simulink model "MDAC3p5bit"  (R2019b)
settings: Solver=VariableStepAuto  StartTime=0.0  StopTime=100.0  RelTol=1e-3
values from neighbouring files (symbols this model uses):
  ts = 1/fs    (= 1)    [launch_pipeline_16ibt.m]
libraries: simulink x1
settings Model: Creator=86184  LastModifiedBy=86184

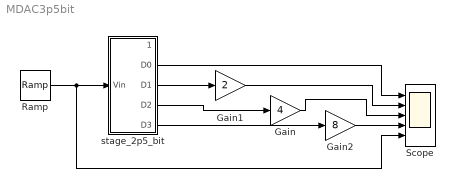
== system MDAC3p5bit ==
  Gain : Gain  Gain=4
  Gain1 : Gain  Gain=2
  Gain2 : Gain  Gain=8
  Ramp : simulink/Sources/Ramp  slope=0.1  start=0  InitialOutput=-5
  Scope : Scope  NumInputPorts=5
  stage_2p5_bit : Subsystem
  wires:
  Ramp/1 -> Scope/5, stage_2p5_bit/1(Vin)
  stage_2p5_bit/2(D0) -> Scope/1
  stage_2p5_bit/3(D1) -> Gain1/1
  stage_2p5_bit/4(D2) -> Gain/1
  Gain1/1 -> Scope/2
  Gain/1 -> Scope/3
  stage_2p5_bit/5(D3) -> Gain2/1
  Gain2/1 -> Scope/4

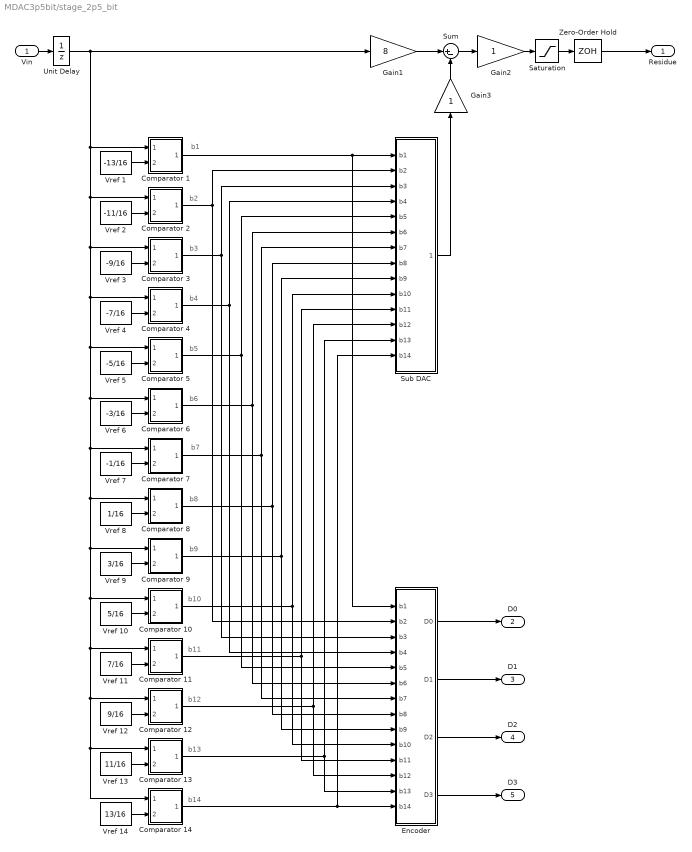
== system MDAC3p5bit/stage_2p5_bit ==
  note: b2
  note: b1
  note: b3
  note: b4
  note: b5
  note: b6
  note: b10
  note: b7
  note: b9
  note: b8
  note: b12
  note: b11
  note: b13
  note: b14
  Vin : Inport
  Comparator 1 : Subsystem
  Comparator 10 : Subsystem
  Comparator 11 : Subsystem
  Comparator 12 : Subsystem
  Comparator 13 : Subsystem
  Comparator 14 : Subsystem
  Comparator 2 : Subsystem
  Comparator 3 : Subsystem
  Comparator 4 : Subsystem
  Comparator 5 : Subsystem
  Comparator 6 : Subsystem
  Comparator 7 : Subsystem
  Comparator 8 : Subsystem
  Comparator 9 : Subsystem
  Encoder : Subsystem
  Gain1 : Gain  Gain=8
  Gain2 : Gain
  Gain3 : Gain
  Saturation : Saturate  UpperLimit=1  LowerLimit=-1
  Sub DAC : Subsystem
  Sum : Sum  Inputs=|+-
  Unit Delay : UnitDelay  SampleTime=-1  HasFrameUpgradeWarning=on
  Vref 1 : Constant  Value=-13/16
  Vref 10 : Constant  Value=5/16
  Vref 11 : Constant  Value=7/16
  Vref 12 : Constant  Value=9/16
  Vref 13 : Constant  Value=11/16
  Vref 14 : Constant  Value=13/16
  Vref 2 : Constant  Value=-11/16
  Vref 3 : Constant  Value=-9/16
  Vref 4 : Constant  Value=-7/16
  Vref 5 : Constant  Value=-5/16
  Vref 6 : Constant  Value=-3/16
  Vref 7 : Constant  Value=-1/16
  Vref 8 : Constant  Value=1/16
  Vref 9 : Constant  Value=3/16
  Zero-Order Hold : ZeroOrderHold  SampleTime=ts
  Residue : Outport
  D0 : Outport  Port=2
  D1 : Outport  Port=3
  D2 : Outport  Port=4
  D3 : Outport  Port=5
  wires:
  Vref 1/1 -> Comparator 1/2(Vref)
  Sub DAC/1(Vdac) -> Gain3/1
  Gain1/1 -> Sum/1
  Gain3/1 -> Sum/2
  Sum/1 -> Gain2/1
  Saturation/1 -> Zero-Order Hold/1
  Zero-Order Hold/1 -> Residue/1
  Gain2/1 -> Saturation/1
  Vref 2/1 -> Comparator 2/2(Vref)
  Vin/1 -> Unit Delay/1
  Vref 3/1 -> Comparator 3/2(Vref)
  Vref 4/1 -> Comparator 4/2(Vref)
  Vref 5/1 -> Comparator 5/2(Vref)
  Vref 6/1 -> Comparator 6/2(Vref)
  Unit Delay/1 -> Comparator 14/1(Vin), Comparator 13/1(Vin), Comparator 12/1(Vin), Comparator 11/1(Vin), Comparator 10/1(Vin), Comparator 9/1(Vin), Comparator 8/1(Vin), Comparator 7/1(Vin), Comparator 6/1(Vin), Comparator 5/1(Vin), Comparator 4/1(Vin), Comparator 3/1(Vin), Comparator 2/1(Vin), Comparator 1/1(Vin), Gain1/1
  Vref 11/1 -> Comparator 11/2(Vref)
  Vref 9/1 -> Comparator 9/2(Vref)
  Vref 7/1 -> Comparator 7/2(Vref)
  Vref 12/1 -> Comparator 12/2(Vref)
  Vref 10/1 -> Comparator 10/2(Vref)
  Vref 8/1 -> Comparator 8/2(Vref)
  Vref 14/1 -> Comparator 14/2(Vref)
  Vref 13/1 -> Comparator 13/2(Vref)
  Comparator 1/1(Out) -> Sub DAC/1(b1), Encoder/1(b1)
  Comparator 2/1(Out) -> Encoder/2(b2), Sub DAC/2(b2)
  Comparator 3/1(Out) -> Encoder/3(b3), Sub DAC/3(b3)
  Comparator 4/1(Out) -> Encoder/4(b4), Sub DAC/4(b4)
  Comparator 5/1(Out) -> Encoder/5(b5), Sub DAC/5(b5)
  Comparator 6/1(Out) -> Encoder/6(b6), Sub DAC/6(b6)
  Comparator 7/1(Out) -> Encoder/7(b7), Sub DAC/7(b7)
  Comparator 8/1(Out) -> Encoder/8(b8), Sub DAC/8(b8)
  Comparator 9/1(Out) -> Encoder/9(b9), Sub DAC/9(b9)
  Comparator 10/1(Out) -> Encoder/10(b10), Sub DAC/10(b10)
  Comparator 11/1(Out) -> Encoder/11(b11), Sub DAC/11(b11)
  Comparator 12/1(Out) -> Encoder/12(b12), Sub DAC/12(b12)
  Comparator 13/1(Out) -> Encoder/13(b13), Sub DAC/13(b13)
  Comparator 14/1(Out) -> Encoder/14(b14), Sub DAC/14(b14)
  Encoder/4(D3) -> D3/1
  Encoder/3(D2) -> D2/1
  Encoder/2(D1) -> D1/1
  Encoder/1(D0) -> D0/1

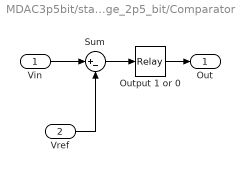
== system MDAC3p5bit/stage_2p5_bit/Comparator 1 ==
  Vin : Inport
  Vref : Inport  Port=2
  Output 1 or 0 : Relay  OnSwitchValue=0  OffSwitchValue=0
  Sum : Sum  Inputs=|+-
  Out : Outport
  wires:
  Sum/1 -> Output 1 or 0/1
  Vin/1 -> Sum/1
  Output 1 or 0/1 -> Out/1
  Vref/1 -> Sum/2

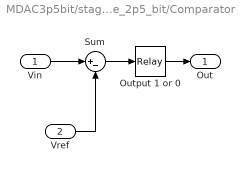
== system MDAC3p5bit/stage_2p5_bit/Comparator 10 ==
  Vin : Inport
  Vref : Inport  Port=2
  Output 1 or 0 : Relay  OnSwitchValue=0  OffSwitchValue=0
  Sum : Sum  Inputs=|+-
  Out : Outport
  wires:
  Sum/1 -> Output 1 or 0/1
  Vin/1 -> Sum/1
  Output 1 or 0/1 -> Out/1
  Vref/1 -> Sum/2

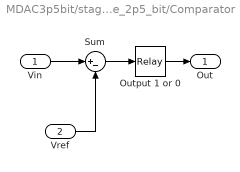
== system MDAC3p5bit/stage_2p5_bit/Comparator 11 ==
  Vin : Inport
  Vref : Inport  Port=2
  Output 1 or 0 : Relay  OnSwitchValue=0  OffSwitchValue=0
  Sum : Sum  Inputs=|+-
  Out : Outport
  wires:
  Sum/1 -> Output 1 or 0/1
  Vin/1 -> Sum/1
  Output 1 or 0/1 -> Out/1
  Vref/1 -> Sum/2

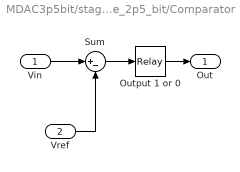
== system MDAC3p5bit/stage_2p5_bit/Comparator 12 ==
  Vin : Inport
  Vref : Inport  Port=2
  Output 1 or 0 : Relay  OnSwitchValue=0  OffSwitchValue=0
  Sum : Sum  Inputs=|+-
  Out : Outport
  wires:
  Sum/1 -> Output 1 or 0/1
  Vin/1 -> Sum/1
  Output 1 or 0/1 -> Out/1
  Vref/1 -> Sum/2

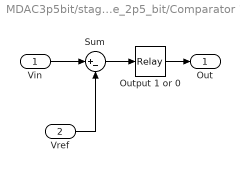
== system MDAC3p5bit/stage_2p5_bit/Comparator 13 ==
  Vin : Inport
  Vref : Inport  Port=2
  Output 1 or 0 : Relay  OnSwitchValue=0  OffSwitchValue=0
  Sum : Sum  Inputs=|+-
  Out : Outport
  wires:
  Sum/1 -> Output 1 or 0/1
  Vin/1 -> Sum/1
  Output 1 or 0/1 -> Out/1
  Vref/1 -> Sum/2

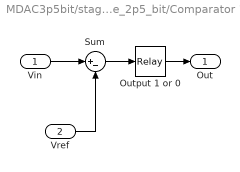
== system MDAC3p5bit/stage_2p5_bit/Comparator 14 ==
  Vin : Inport
  Vref : Inport  Port=2
  Output 1 or 0 : Relay  OnSwitchValue=0  OffSwitchValue=0
  Sum : Sum  Inputs=|+-
  Out : Outport
  wires:
  Sum/1 -> Output 1 or 0/1
  Vin/1 -> Sum/1
  Output 1 or 0/1 -> Out/1
  Vref/1 -> Sum/2

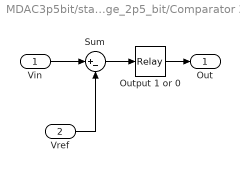
== system MDAC3p5bit/stage_2p5_bit/Comparator 2 ==
  Vin : Inport
  Vref : Inport  Port=2
  Output 1 or 0 : Relay  OnSwitchValue=0  OffSwitchValue=0
  Sum : Sum  Inputs=|+-
  Out : Outport
  wires:
  Sum/1 -> Output 1 or 0/1
  Vin/1 -> Sum/1
  Output 1 or 0/1 -> Out/1
  Vref/1 -> Sum/2

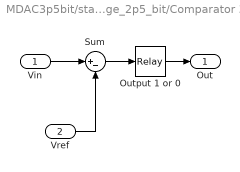
== system MDAC3p5bit/stage_2p5_bit/Comparator 3 ==
  Vin : Inport
  Vref : Inport  Port=2
  Output 1 or 0 : Relay  OnSwitchValue=0  OffSwitchValue=0
  Sum : Sum  Inputs=|+-
  Out : Outport
  wires:
  Sum/1 -> Output 1 or 0/1
  Vin/1 -> Sum/1
  Output 1 or 0/1 -> Out/1
  Vref/1 -> Sum/2

== system MDAC3p5bit/stage_2p5_bit/Comparator 4 ==
  Vin : Inport
  Vref : Inport  Port=2
  Output 1 or 0 : Relay  OnSwitchValue=0  OffSwitchValue=0
  Sum : Sum  Inputs=|+-
  Out : Outport
  wires:
  Sum/1 -> Output 1 or 0/1
  Vin/1 -> Sum/1
  Output 1 or 0/1 -> Out/1
  Vref/1 -> Sum/2

== system MDAC3p5bit/stage_2p5_bit/Comparator 5 ==
  Vin : Inport
  Vref : Inport  Port=2
  Output 1 or 0 : Relay  OnSwitchValue=0  OffSwitchValue=0
  Sum : Sum  Inputs=|+-
  Out : Outport
  wires:
  Sum/1 -> Output 1 or 0/1
  Vin/1 -> Sum/1
  Output 1 or 0/1 -> Out/1
  Vref/1 -> Sum/2

== system MDAC3p5bit/stage_2p5_bit/Comparator 6 ==
  Vin : Inport
  Vref : Inport  Port=2
  Output 1 or 0 : Relay  OnSwitchValue=0  OffSwitchValue=0
  Sum : Sum  Inputs=|+-
  Out : Outport
  wires:
  Sum/1 -> Output 1 or 0/1
  Vin/1 -> Sum/1
  Output 1 or 0/1 -> Out/1
  Vref/1 -> Sum/2

== system MDAC3p5bit/stage_2p5_bit/Comparator 7 ==
  Vin : Inport
  Vref : Inport  Port=2
  Output 1 or 0 : Relay  OnSwitchValue=0  OffSwitchValue=0
  Sum : Sum  Inputs=|+-
  Out : Outport
  wires:
  Sum/1 -> Output 1 or 0/1
  Vin/1 -> Sum/1
  Output 1 or 0/1 -> Out/1
  Vref/1 -> Sum/2

== system MDAC3p5bit/stage_2p5_bit/Comparator 8 ==
  Vin : Inport
  Vref : Inport  Port=2
  Output 1 or 0 : Relay  OnSwitchValue=0  OffSwitchValue=0
  Sum : Sum  Inputs=|+-
  Out : Outport
  wires:
  Sum/1 -> Output 1 or 0/1
  Vin/1 -> Sum/1
  Output 1 or 0/1 -> Out/1
  Vref/1 -> Sum/2

== system MDAC3p5bit/stage_2p5_bit/Comparator 9 ==
  Vin : Inport
  Vref : Inport  Port=2
  Output 1 or 0 : Relay  OnSwitchValue=0  OffSwitchValue=0
  Sum : Sum  Inputs=|+-
  Out : Outport
  wires:
  Sum/1 -> Output 1 or 0/1
  Vin/1 -> Sum/1
  Output 1 or 0/1 -> Out/1
  Vref/1 -> Sum/2

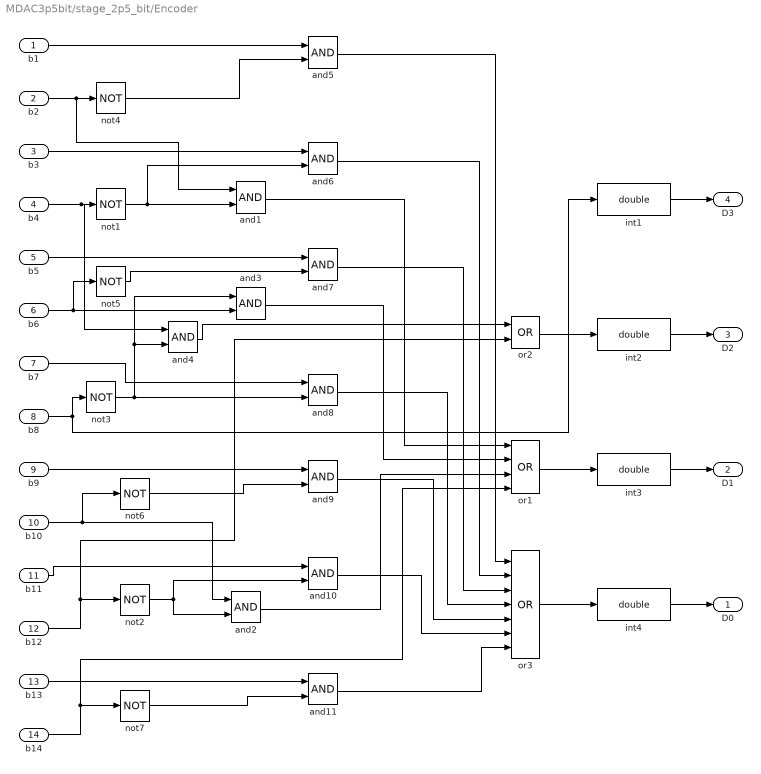
== system MDAC3p5bit/stage_2p5_bit/Encoder ==
  b1 : Inport
  b2 : Inport  Port=2
  b3 : Inport  Port=3
  b4 : Inport  Port=4
  b5 : Inport  Port=5
  b6 : Inport  Port=6
  b7 : Inport  Port=7
  b8 : Inport  Port=8
  b9 : Inport  Port=9
  b10 : Inport  Port=10
  b11 : Inport  Port=11
  b12 : Inport  Port=12
  b13 : Inport  Port=13
  b14 : Inport  Port=14
  and{1..11} (11 alike) : Logic  AllPortsSameDT=off  OutDataTypeStr=boolean
  int{1..4} (4 alike) : DataTypeConversion  OutDataTypeStr=double
  not{1..7} (7 alike) : Logic  Operator=NOT  AllPortsSameDT=off  OutDataTypeStr=boolean
  or1 : Logic  Operator=OR  Inputs=4  AllPortsSameDT=off  OutDataTypeStr=boolean
  or2 : Logic  Operator=OR  AllPortsSameDT=off  OutDataTypeStr=boolean
  or3 : Logic  Operator=OR  Inputs=7  AllPortsSameDT=off  OutDataTypeStr=boolean
  D0 : Outport
  D1 : Outport  Port=2
  D2 : Outport  Port=3
  D3 : Outport  Port=4
  wires:
  int3/1 -> D1/1
  int4/1 -> D0/1
  int2/1 -> D2/1
  int1/1 -> D3/1
  b8/1 -> not3/1, int1/1
  b4/1 -> and4/1, not1/1
  not3/1 -> and3/1, and4/2, and8/2
  and4/1 -> or2/1
  b12/1 -> not2/1, or2/2
  b2/1 -> not4/1, and1/1
  not1/1 -> and6/2, and1/2
  b6/1 -> not5/1, and3/2
  b10/1 -> not6/1, and2/1
  not2/1 -> and2/2, and10/2
  b14/1 -> not7/1, or1/4
  and2/1 -> or1/3
  and3/1 -> or1/2
  and1/1 -> or1/1
  or2/1 -> int2/1
  or1/1 -> int3/1
  b1/1 -> and5/1
  not4/1 -> and5/2
  b3/1 -> and6/1
  b5/1 -> and7/1
  not5/1 -> and7/2
  b7/1 -> and8/1
  b9/1 -> and9/1
  not6/1 -> and9/2
  b11/1 -> and10/1
  b13/1 -> and11/1
  not7/1 -> and11/2
  or3/1 -> int4/1
  and5/1 -> or3/1
  and6/1 -> or3/2
  and7/1 -> or3/3
  and8/1 -> or3/4
  and9/1 -> or3/5
  and10/1 -> or3/6
  and11/1 -> or3/7

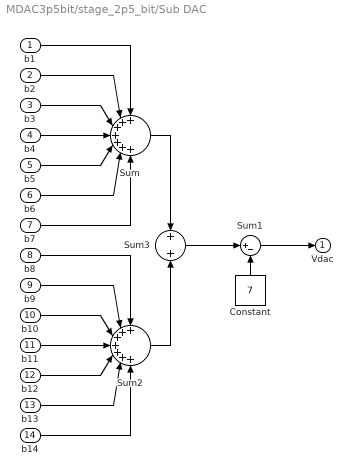
== system MDAC3p5bit/stage_2p5_bit/Sub DAC ==
  b1 : Inport
  b2 : Inport  Port=2
  b3 : Inport  Port=3
  b4 : Inport  Port=4
  b5 : Inport  Port=5
  b6 : Inport  Port=6
  b7 : Inport  Port=7
  b8 : Inport  Port=8
  b9 : Inport  Port=9
  b10 : Inport  Port=10
  b11 : Inport  Port=11
  b12 : Inport  Port=12
  b13 : Inport  Port=13
  b14 : Inport  Port=14
  Constant : Constant  Value=7
  Sum : Sum  Inputs=+++++++
  Sum1 : Sum  Inputs=|+-
  Sum2 : Sum  Inputs=+++++++
  Sum3 : Sum
  Vdac : Outport
  wires:
  b1/1 -> Sum/1
  b2/1 -> Sum/2
  b3/1 -> Sum/3
  b4/1 -> Sum/4
  b5/1 -> Sum/5
  b6/1 -> Sum/6
  Constant/1 -> Sum1/2
  b7/1 -> Sum/7
  Sum/1 -> Sum3/1
  Sum3/1 -> Sum1/1
  Sum1/1 -> Vdac/1
  b8/1 -> Sum2/1
  b9/1 -> Sum2/2
  b12/1 -> Sum2/5
  b13/1 -> Sum2/6
  b10/1 -> Sum2/3
  b11/1 -> Sum2/4
  b14/1 -> Sum2/7
  Sum2/1 -> Sum3/2
